simulink model "HLSDem_SetPoint"  (R2016b)
settings: configuration reference "CodeGenConfigSet" (kept outside this file)
values from neighbouring files (symbols this model uses):
  EPM_N_MAX = fi(10000,EngSpeed_rpm)    [init_HLSDem_SetPoint.m]    (also in init_HLSDem_SetPoint_SIL.m)
  HLSDem_dnSetPLoLimHiTrm_C = Calibration.Parameter    [init_HLSDem_SetPoint.m]    (also in init_HLSDem_SetPoint_SIL.m = Simulink.Parameter)
  HLSDem_dnSetPLoLimLoTrm_C = Calibration.Parameter    [init_HLSDem_SetPoint.m]    (also in init_HLSDem_SetPoint_SIL.m = Simulink.Parameter)
  HLSDem_facFdbkCANKick_C = Calibration.Parameter    [init_HLSDem_SetPoint.m]    (also in init_HLSDem_SetPoint_SIL.m = Simulink.Parameter)
  HLSDem_facFdbkDrvKick_C = Calibration.Parameter    [init_HLSDem_SetPoint.m]    (also in init_HLSDem_SetPoint_SIL.m = Simulink.Parameter)
  HLSDem_facFdbkHGG_C = Calibration.Parameter    [init_HLSDem_SetPoint.m]    (also in init_HLSDem_SetPoint_SIL.m = Simulink.Parameter)
  HLSDem_facFdbkLGG_C = Calibration.Parameter    [init_HLSDem_SetPoint.m]    (also in init_HLSDem_SetPoint_SIL.m = Simulink.Parameter)
  HLSDem_facFdbkMaxAcs_C = Calibration.Parameter    [init_HLSDem_SetPoint.m]    (also in init_HLSDem_SetPoint_SIL.m = Simulink.Parameter)
  HLSDem_facFdbkMaxSysErr_C = Calibration.Parameter    [init_HLSDem_SetPoint.m]    (also in init_HLSDem_SetPoint_SIL.m = Simulink.Parameter)
  HLSDem_facFdbkMaxTra_C = Calibration.Parameter    [init_HLSDem_SetPoint.m]    (also in init_HLSDem_SetPoint_SIL.m = Simulink.Parameter)
  HLSDem_facFdbkRed1_C = Calibration.Parameter    [init_HLSDem_SetPoint.m]    (also in init_HLSDem_SetPoint_SIL.m = Simulink.Parameter)
  HLSDem_facFdbkRed2_C = Calibration.Parameter    [init_HLSDem_SetPoint.m]    (also in init_HLSDem_SetPoint_SIL.m = Simulink.Parameter)
  HLSDem_facFdbkRed3_C = Calibration.Parameter    [init_HLSDem_SetPoint.m]    (also in init_HLSDem_SetPoint_SIL.m = Simulink.Parameter)
  HLSDem_facFdbkStrt_C = Calibration.Parameter    [init_HLSDem_SetPoint.m]    (also in init_HLSDem_SetPoint_SIL.m = Simulink.Parameter)
  HLSDem_facFdbkSysDgrt1_C = Calibration.Parameter    [init_HLSDem_SetPoint.m]    (also in init_HLSDem_SetPoint_SIL.m = Simulink.Parameter)
  HLSDem_facFdbkSysDgrt2_C = Calibration.Parameter    [init_HLSDem_SetPoint.m]    (also in init_HLSDem_SetPoint_SIL.m = Simulink.Parameter)
  HLSDem_facFdbkSysDgrt3_C = Calibration.Parameter    [init_HLSDem_SetPoint.m]    (also in init_HLSDem_SetPoint_SIL.m = Simulink.Parameter)
  HLSDem_facSetPLoFlt_C = Calibration.Parameter    [init_HLSDem_SetPoint.m]    (also in init_HLSDem_SetPoint_SIL.m = Simulink.Parameter)
  HLSDem_facTrqHiPT1_C = Calibration.Parameter    [init_HLSDem_SetPoint.m]    (also in init_HLSDem_SetPoint_SIL.m = Simulink.Parameter)
  HLSDem_facTrqLoPT1_C = Calibration.Parameter    [init_HLSDem_SetPoint.m]    (also in init_HLSDem_SetPoint_SIL.m = Simulink.Parameter)
  HLSDem_nHGGSetPHi_C = Calibration.Parameter    [init_HLSDem_SetPoint.m]    (also in init_HLSDem_SetPoint_SIL.m = Simulink.Parameter)
  HLSDem_nKDSetPHi_C = Calibration.Parameter    [init_HLSDem_SetPoint.m]    (also in init_HLSDem_SetPoint_SIL.m = Simulink.Parameter)
  HLSDem_nLGGSetPHi_C = Calibration.Parameter    [init_HLSDem_SetPoint.m]    (also in init_HLSDem_SetPoint_SIL.m = Simulink.Parameter)
  HLSDem_nRed1SetPHi_C = Calibration.Parameter    [init_HLSDem_SetPoint.m]    (also in init_HLSDem_SetPoint_SIL.m = Simulink.Parameter)
  HLSDem_nRed2SetPHi_C = Calibration.Parameter    [init_HLSDem_SetPoint.m]    (also in init_HLSDem_SetPoint_SIL.m = Simulink.Parameter)
  HLSDem_nRed3SetPHi_C = Calibration.Parameter    [init_HLSDem_SetPoint.m]    (also in init_HLSDem_SetPoint_SIL.m = Simulink.Parameter)
  HLSDem_nSel1SetPLo_C = Calibration.Parameter    [init_HLSDem_SetPoint.m]    (also in init_HLSDem_SetPoint_SIL.m = Simulink.Parameter)
  HLSDem_nSel2SetPLo_C = Calibration.Parameter    [init_HLSDem_SetPoint.m]    (also in init_HLSDem_SetPoint_SIL.m = Simulink.Parameter)
  HLSDem_nSel3SetPLo_C = Calibration.Parameter    [init_HLSDem_SetPoint.m]    (also in init_HLSDem_SetPoint_SIL.m = Simulink.Parameter)
  HLSDem_nSetPLoDia_C = Calibration.Parameter    [init_HLSDem_SetPoint.m]    (also in init_HLSDem_SetPoint_SIL.m = Simulink.Parameter)
  HLSDem_nSetPLoDrvAwy_C = Calibration.Parameter    [init_HLSDem_SetPoint.m]    (also in init_HLSDem_SetPoint_SIL.m = Simulink.Parameter)
  HLSDem_nSetPLoIni_CUR = Calibration.Parameter    [init_HLSDem_SetPoint.m]    (also in init_HLSDem_SetPoint_SIL.m = Simulink.Parameter)
  HLSDem_nSetPLoIni_CURX = Calibration.Parameter    [init_HLSDem_SetPoint.m]    (also in init_HLSDem_SetPoint_SIL.m = Simulink.Parameter)
  HLSDem_nSetPLoMax_C = Calibration.Parameter    [init_HLSDem_SetPoint.m]    (also in init_HLSDem_SetPoint_SIL.m = Simulink.Parameter)
  HLSDem_nSetPLoMaxOfs_C = Calibration.Parameter    [init_HLSDem_SetPoint.m]    (also in init_HLSDem_SetPoint_SIL.m = Simulink.Parameter)
  HLSDem_nSetPLoOfsMoF_C = Calibration.Parameter    [init_HLSDem_SetPoint.m]    (also in init_HLSDem_SetPoint_SIL.m = Simulink.Parameter)
  HLSDem_nSetPLoWrm_C = Calibration.Parameter    [init_HLSDem_SetPoint.m]    (also in init_HLSDem_SetPoint_SIL.m = Simulink.Parameter)
  HLSDem_nSpdLowBattUAdd_CUR = Calibration.Parameter    [init_HLSDem_SetPoint.m]    (also in init_HLSDem_SetPoint_SIL.m = Simulink.Parameter)
  HLSDem_nSpdLowBattUAdd_CURX = Calibration.Parameter    [init_HLSDem_SetPoint.m]    (also in init_HLSDem_SetPoint_SIL.m = Simulink.Parameter)
  HLSDem_nSpdLowBattUAddLim_C = Calibration.Parameter    [init_HLSDem_SetPoint.m]    (also in init_HLSDem_SetPoint_SIL.m = Simulink.Parameter)
  HLSDem_nStrtSetPHi_C = Calibration.Parameter    [init_HLSDem_SetPoint.m]    (also in init_HLSDem_SetPoint_SIL.m = Simulink.Parameter)
  HLSDem_nSysDgrtSetPHi_C = Calibration.Parameter    [init_HLSDem_SetPoint.m]    (also in init_HLSDem_SetPoint_SIL.m = Simulink.Parameter)
  HLSDem_rTrqSwt_C = Calibration.Parameter    [init_HLSDem_SetPoint.m]    (also in init_HLSDem_SetPoint_SIL.m = Simulink.Parameter)
  HLSDem_SetPHiRmpSlopeNeg_C = Calibration.Parameter    [init_HLSDem_SetPoint.m]    (also in init_HLSDem_SetPoint_SIL.m = Simulink.Parameter)
  HLSDem_SetPHiRmpSlopePos_C = Calibration.Parameter    [init_HLSDem_SetPoint.m]    (also in init_HLSDem_SetPoint_SIL.m = Simulink.Parameter)
  HLSDem_SetPLoRmpSlopeNeg_C = Calibration.Parameter    [init_HLSDem_SetPoint.m]    (also in init_HLSDem_SetPoint_SIL.m = Simulink.Parameter)
  HLSDem_SetPLoRmpSlopePos_C = Calibration.Parameter    [init_HLSDem_SetPoint.m]    (also in init_HLSDem_SetPoint_SIL.m = Simulink.Parameter)
  HLSDem_SetPLoTipInRmpSlopeNeg_C = Calibration.Parameter    [init_HLSDem_SetPoint.m]    (also in init_HLSDem_SetPoint_SIL.m = Simulink.Parameter)
  HLSDem_SetPLoTipInRmpSlopePos_C = Calibration.Parameter    [init_HLSDem_SetPoint.m]    (also in init_HLSDem_SetPoint_SIL.m = Simulink.Parameter)
  HLSDem_stSetPLoFlt_C = Calibration.Parameter    [init_HLSDem_SetPoint.m]    (also in init_HLSDem_SetPoint_SIL.m = Simulink.Parameter)
  HLSDem_stSpdSel_C = Calibration.Parameter    [init_HLSDem_SetPoint.m]    (also in init_HLSDem_SetPoint_SIL.m = Simulink.Parameter)
  HLSDem_stSysDgrtSetPHi_C = Calibration.Parameter    [init_HLSDem_SetPoint.m]    (also in init_HLSDem_SetPoint_SIL.m = Simulink.Parameter)
  HLSDem_swtDisblVehIfcSetPHi_C = Calibration.Parameter    [init_HLSDem_SetPoint.m]    (also in init_HLSDem_SetPoint_SIL.m = Simulink.Parameter)
  HLSDem_swtEnaPTO_C = Calibration.Parameter    [init_HLSDem_SetPoint.m]    (also in init_HLSDem_SetPoint_SIL.m = Simulink.Parameter)
  HLSDem_swtMode_C = Calibration.Parameter    [init_HLSDem_SetPoint.m]    (also in init_HLSDem_SetPoint_SIL.m = Simulink.Parameter)
  HLSDem_swtTempSel_C = Calibration.Parameter    [init_HLSDem_SetPoint.m]    (also in init_HLSDem_SetPoint_SIL.m = Simulink.Parameter)
  HLSDem_swtTrqHiSel_C = Calibration.Parameter    [init_HLSDem_SetPoint.m]    (also in init_HLSDem_SetPoint_SIL.m = Simulink.Parameter)
  HLSDem_swtTrqLoSel_C = Calibration.Parameter    [init_HLSDem_SetPoint.m]    (also in init_HLSDem_SetPoint_SIL.m = Simulink.Parameter)
  HLSDem_tDflSetPLo_C = Calibration.Parameter    [init_HLSDem_SetPoint.m]    (also in init_HLSDem_SetPoint_SIL.m = Simulink.Parameter)
  HLSDem_tiMaxIncrSetPLo_C = Calibration.Parameter    [init_HLSDem_SetPoint.m]    (also in init_HLSDem_SetPoint_SIL.m = Simulink.Parameter)
  HLSDem_tiSpdLowBattUAdd_C = Calibration.Parameter    [init_HLSDem_SetPoint.m]    (also in init_HLSDem_SetPoint_SIL.m = Simulink.Parameter)
  HLSDem_tiStrtCEngDsT_CUR = Calibration.Parameter    [init_HLSDem_SetPoint.m]    (also in init_HLSDem_SetPoint_SIL.m = Simulink.Parameter)
  HLSDem_tiStrtCEngDsT_CURX = Calibration.Parameter    [init_HLSDem_SetPoint.m]    (also in init_HLSDem_SetPoint_SIL.m = Simulink.Parameter)
  HLSDem_tiStrtEngOil_CUR = Calibration.Parameter    [init_HLSDem_SetPoint.m]    (also in init_HLSDem_SetPoint_SIL.m = Simulink.Parameter)
  HLSDem_tiStrtEngOil_CURX = Calibration.Parameter    [init_HLSDem_SetPoint.m]    (also in init_HLSDem_SetPoint_SIL.m = Simulink.Parameter)
  HLSDem_tThresDisbl_C = Calibration.Parameter    [init_HLSDem_SetPoint.m]    (also in init_HLSDem_SetPoint_SIL.m = Simulink.Parameter)
  HLSDem_tThresEna_C = Calibration.Parameter    [init_HLSDem_SetPoint.m]    (also in init_HLSDem_SetPoint_SIL.m = Simulink.Parameter)
  HLSDem_volSpdAddHi_C = Calibration.Parameter    [init_HLSDem_SetPoint.m]    (also in init_HLSDem_SetPoint_SIL.m = Simulink.Parameter)
  HLSDem_volSpdAddLo_C = Calibration.Parameter    [init_HLSDem_SetPoint.m]    (also in init_HLSDem_SetPoint_SIL.m = Simulink.Parameter)
  HndBrk_stDebVal_C = Calibration.Parameter    [init_HLSDem_SetPoint.m]    (also in init_HLSDem_SetPoint_SIL.m = Simulink.Parameter)
  SigTst_nSetPHi_C = Calibration.Parameter    [init_HLSDem_SetPoint.m]    (also in init_HLSDem_SetPoint_SIL.m = Simulink.Parameter)
  SigTst_nSetPLo_C = Calibration.Parameter    [init_HLSDem_SetPoint.m]    (also in init_HLSDem_SetPoint_SIL.m = Simulink.Parameter)
  SigTst_swtSetPHi_C = Calibration.Parameter    [init_HLSDem_SetPoint.m]    (also in init_HLSDem_SetPoint_SIL.m = Simulink.Parameter)
  SigTst_swtSetPLo_C = Calibration.Parameter    [init_HLSDem_SetPoint.m]    (also in init_HLSDem_SetPoint_SIL.m = Simulink.Parameter)
undefined symbols (not defined in the file or in its folder): CEngDst_switch_conv, CEngDsT_tTransf_CURX, EngState_conv, HLSDem_SetPoint_DT, StSys_StrtState_conv, Switch_conv
libraries: CXLib x13, simulink x3
(part 2 of 2)

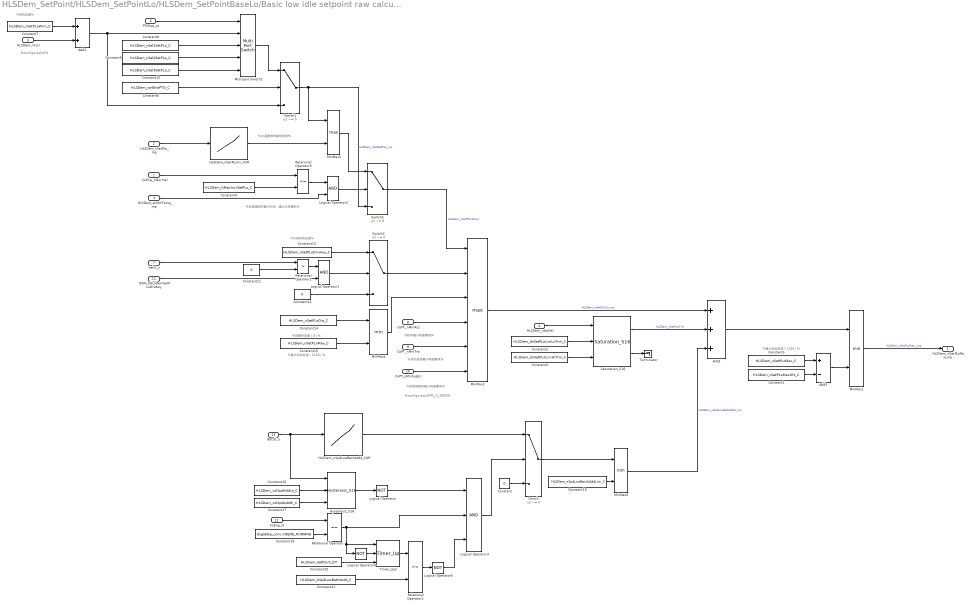
== system HLSDem_SetPoint/HLSDem_SetPointLo/HLSDem_SetPointBaseLo/Basic low idle setpoint raw calculation ==
  note: %最大目标怠速（1100）%
  note: %故障时怠速（0）%
  note: %configured=EPM_N_ZERO%
  note: %怠速增加的最大时间，确认已经暖机%
  note: %热机怠速%
  note: %最大目标怠速（1100）%
  note: %行驶时的怠速%
  note: %附件最小转速需求%
  note: %系统错误时最小转速需求%
  note: %传动系统最小转速需求%
  note: %configured=0%
  note: %水温要求的最低转速%
  CoEng_tiNormal : Inport
  HLSDem_tSetPLo_mp : Inport  Port=2
  HLSDem_stStrtTemp_mp : Inport  Port=3
  HLSDem_nAdjVal : Inport  Port=4
  HLSDem_nIncr : Inport  Port=5
  PTOSwt_st : Inport  Port=6
  VehV_v : Inport  Port=7
  CoPT_nMinAcs : Inport  Port=8
  CoPT_nMinTra : Inport  Port=9
  CoPT_nMinSysErr : Inport  Port=10
  DSM_bHLSDemSetPLoDrvAwy : Inport  Port=11
  CoEng_st : Inport  Port=12
  BattU_u : Inport  Tag=mv  Description=Battery voltage  Port=13  OutMin=0  OutMax=50000  OutDataTypeStr=Battery_mv
  Add1 : Sum  Inputs=+++  SaturateOnIntegerOverflow=on  InputSameDT=on
  Add2 : Sum  SaturateOnIntegerOverflow=on  InputSameDT=on
  Add3 : Sum  Inputs=+-  SaturateOnIntegerOverflow=on  InputSameDT=on
  Constant : Constant  Value=0  OutDataTypeStr=Inherit: Inherit via back propagation
  Constant1 : Constant  Value=HLSDem_nSetPLoMaxOfs_C
  Constant10 : Constant  Value=HLSDem_nSel3SetPLo_C
  Constant11 : Constant  Value=0  OutDataTypeStr=Inherit: Inherit via back propagation
  Constant12 : Constant  Value=0  OutDataTypeStr=Inherit: Inherit via back propagation
  Constant13 : Constant  Value=HLSDem_nSetPLoDrvAwy_C
  Constant14 : Constant  Value=HLSDem_nSetPLoDia_C
  Constant15 : Constant  Value=HLSDem_nSetPLoMax_C
  Constant16 : Constant  Value=HLSDem_volSpdAddLo_C
  Constant17 : Constant  Value=HLSDem_volSpdAddHi_C
  Constant18 : Constant  Value=EngState_conv.COENG_RUNNING
  Constant19 : Constant  Value=HLSDem_nSpdLowBattUAddLim_C
  Constant2 : Constant  Value=HLSDem_dnSetPLoLimLoTrm_C  SampleTime=-1
  Constant20 : Constant  Value=HLSDem_SetPoint_DT  OutDataTypeStr=Inherit: Inherit via back propagation
  Constant21 : Constant  Value=HLSDem_tiSpdLowBattUAdd_C
  Constant3 : Constant  Value=HLSDem_dnSetPLoLimHiTrm_C  SampleTime=-1
  Constant4 : Constant  Value=HLSDem_tiMaxIncrSetPLo_C
  Constant5 : Constant  Value=HLSDem_nSetPLoMax_C
  Constant6 : Constant  Value=HLSDem_swtEnaPTO_C
  Constant7 : Constant  Value=HLSDem_nSetPLoWrm_C
  Constant8 : Constant  Value=HLSDem_nSel1SetPLo_C
  Constant9 : Constant  Value=HLSDem_nSel2SetPLo_C
  HLSDem_nSetPLoIni_CUR : Lookup_n-D  DialogController=Simulink.DDGSource  NumberOfTableDimensions=1  BreakpointsForDimension1=HLSDem_nSetPLoIni_CURX  BreakpointsForDimension2=CEngDsT_tTransf_CURX  IndexSearchMethod=Linear search  BeginIndexSearchUsingPreviousIndexResult=on  Table=HLSDem_nSetPLoIni_CUR  ExtrapMethod=Clip  UseLastTableValue=on  InternalRulePriority=Speed  OutDataTypeStr=Inherit: Inherit via back propagation  SaturateOnIntegerOverflow=on
  HLSDem_nSpdLowBattUAdd_CUR : Lookup_n-D  NumberOfTableDimensions=1  BreakpointsForDimension1=HLSDem_nSpdLowBattUAdd_CURX  IndexSearchMethod=Linear search  BeginIndexSearchUsingPreviousIndexResult=on  Table=HLSDem_nSpdLowBattUAdd_CUR  ExtrapMethod=Clip  UseLastTableValue=on  InternalRulePriority=Speed  OutDataTypeStr=Inherit: Inherit from 'Table data'  RndMeth=Simplest  SaturateOnIntegerOverflow=on
  Hysteresis_S16 : CXLib/Hysteresis_S16
  Logical Operator : Logic  Operator=NOT  AllPortsSameDT=off  OutDataTypeStr=boolean
  Logical Operator1 : Logic  OutDataTypeStr=boolean
  Logical Operator2 : Logic  OutDataTypeStr=boolean
  Logical Operator3 : Logic  Inputs=3  AllPortsSameDT=off  OutDataTypeStr=boolean
  Logical Operator4 : Logic  Operator=NOT  AllPortsSameDT=off  OutDataTypeStr=boolean
  Logical Operator5 : Logic  Operator=NOT  AllPortsSameDT=off  OutDataTypeStr=boolean
  MinMax1 : MinMax  Inputs=2  SaturateOnIntegerOverflow=on  InputSameDT=on
  MinMax2 : MinMax  RequirementInfo={'other' 'HLSDem_SetPointLo_requirements.docx' '@Simulink_requirement_item_20' 'true' '选择目标怠速' '' } %GIDa_1dec2fce_e581_44b4_8998_b8679ade50a4  Function=max  Inputs=6  SaturateOnIntegerOverflow=on  InputSameDT=on
  MinMax3 : MinMax  Function=max  Inputs=2  SaturateOnIntegerOverflow=on  InputSameDT=on
  MinMax4 : MinMax  Inputs=2  SaturateOnIntegerOverflow=on  InputSameDT=on
  MinMax5 : MinMax  Inputs=2  SaturateOnIntegerOverflow=on
  Multiport Switch2 : MultiPortSwitch  DataPortOrder=Zero-based contiguous  Inputs=4  DiagnosticForDefault=Warning  SaturateOnIntegerOverflow=on  InputSameDT=on
  Relational Operator : RelationalOperator  Operator===  OutDataTypeStr=boolean  RndMeth=Simplest
  Relational Operator1 : RelationalOperator  Operator=>  OutDataTypeStr=boolean  RndMeth=Nearest  InputSameDT=on
  Relational Operator2 : RelationalOperator  OutDataTypeStr=boolean  RndMeth=Simplest  InputSameDT=on
  Relational Operator9 : RelationalOperator  Operator=<=  OutDataTypeStr=boolean  RndMeth=Nearest  InputSameDT=on
  Saturation_S16 : CXLib/Saturation_S16  RequirementInfo={'other' 'HLSDem_SetPointLo_requirements.docx' '@Simulink_requirement_item_21' 'true' '目标怠速调整及限制' '' } %GIDa_15563632_a417_4a1b_8a84_0934a39ef2cd
  Switch : Switch  Criteria=u2 ~= 0  InputSameDT=on
  Switch1 : Switch  Criteria=u2 ~= 0  SaturateOnIntegerOverflow=on  InputSameDT=on
  Switch2 : Switch  Criteria=u2 ~= 0  SaturateOnIntegerOverflow=on  InputSameDT=on
  Switch5 : Switch  RequirementInfo={'other' 'HLSDem_SetPointLo_requirements.docx' '@Simulink_requirement_item_19' 'true' '目标怠速自动增加功能' '' } %GIDa_4e10bb43_f23f_486a_82bf_1b96970b13ef  Criteria=u2 ~= 0  SaturateOnIntegerOverflow=on  InputSameDT=on
  Terminator : Terminator
  Timer_Up2 : CXLib/Timer_Up
  HLSDem_nSetPLoRaw_mp : Outport
  wires:
  Constant11/1 -> Relational Operator1/2
  CoPT_nMinSysErr/1 -> MinMax2/6
  CoPT_nMinTra/1 -> MinMax2/5
  CoPT_nMinAcs/1 -> MinMax2/4
  MinMax4/1 -> MinMax2/3
  Constant15/1 -> MinMax4/2
  Constant14/1 -> MinMax4/1
  Switch2/1 -> MinMax2/2
  Constant13/1 -> Switch2/1
  Constant12/1 -> Switch2/3
  DSM_bHLSDemSetPLoDrvAwy/1 -> Logical Operator1/2
  Relational Operator1/1 -> Logical Operator1/1
  VehV_v/1 -> Relational Operator1/1
  Logical Operator1/1 -> Switch2/2
  Switch5/1 -> MinMax2/1  "HLSDem_nSetPLoTemp"
  MinMax3/1 -> Switch5/1
  Constant10/1 -> Multiport Switch2/5
  Constant9/1 -> Multiport Switch2/4
  Constant8/1 -> Multiport Switch2/3
  PTOSwt_st/1 -> Multiport Switch2/1
  Multiport Switch2/1 -> Switch1/1
  HLSDem_nIncr/1 -> Add2/2
  Constant7/1 -> Add2/1
  Add2/1 -> Multiport Switch2/2, Switch1/3
  Constant6/1 -> Switch1/2
  Switch1/1 -> MinMax3/1, Switch5/3  "HLSDem_nSelSetPLo_mp"
  HLSDem_tSetPLo_mp/1 -> HLSDem_nSetPLoIni_CUR/1
  HLSDem_nSetPLoIni_CUR/1 -> MinMax3/2
  HLSDem_stStrtTemp_mp/1 -> Logical Operator2/2
  CoEng_tiNormal/1 -> Relational Operator9/1
  Constant4/1 -> Relational Operator9/2
  Relational Operator9/1 -> Logical Operator2/1
  Logical Operator2/1 -> Switch5/2
  MinMax2/1 -> Add1/1  "HLSDem_nSetPLoCo_mp"
  HLSDem_nAdjVal/1 -> Saturation_S16/1
  Constant3/1 -> Saturation_S16/3
  Constant2/1 -> Saturation_S16/2
  Saturation_S16/2 -> Terminator/1
  Saturation_S16/1 -> Add1/2  "HLSDem_nSetPLoTrm"
  Add1/1 -> MinMax1/1
  MinMax1/1 -> HLSDem_nSetPLoRaw_mp/1  "HLSDem_nSetPLoRaw_mp"
  Constant1/1 -> Add3/2
  Constant5/1 -> Add3/1
  Add3/1 -> MinMax1/2
  BattU_u/1 -> Hysteresis_S16/1, HLSDem_nSpdLowBattUAdd_CUR/1
  HLSDem_nSpdLowBattUAdd_CUR/1 -> Switch/1
  Hysteresis_S16/1 -> Logical Operator/1
  Constant/1 -> Switch/3
  Constant16/1 -> Hysteresis_S16/2
  Constant17/1 -> Hysteresis_S16/3
  CoEng_st/1 -> Relational Operator/1
  Constant18/1 -> Relational Operator/2
  Logical Operator/1 -> Logical Operator3/1
  Relational Operator/1 -> Logical Operator3/2, Timer_Up2/1, Logical Operator4/1
  Logical Operator3/1 -> Switch/2
  Switch/1 -> MinMax5/1
  MinMax5/1 -> Add1/3  "HLSDem_nSpdLowBattUAdd_mp"
  Constant19/1 -> MinMax5/2
  Logical Operator4/1 -> Timer_Up2/2
  Constant20/1 -> Timer_Up2/3
  Timer_Up2/1 -> Relational Operator2/1
  Constant21/1 -> Relational Operator2/2
  Relational Operator2/1 -> Logical Operator5/1
  Logical Operator5/1 -> Logical Operator3/3

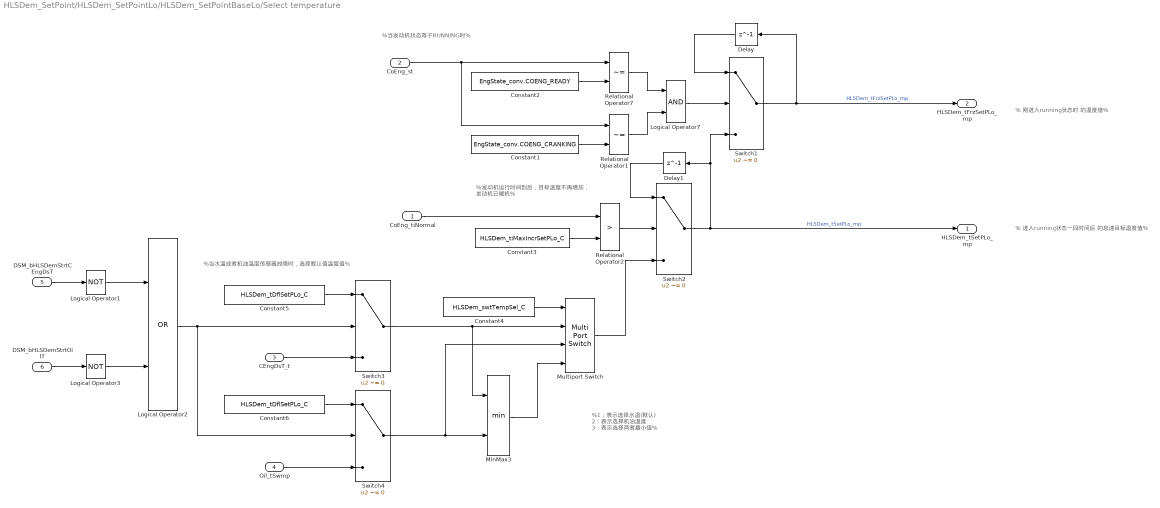
== system HLSDem_SetPoint/HLSDem_SetPointLo/HLSDem_SetPointBaseLo/Select temperature ==
  note: %当水温或者机油温度传感器故障时，选择默认值温度值%
  note: %当发动机状态等于RUNNING时%
  note: % 刚进入running状态时 的温度值%
  note: % 进入running状态一段时间后 的怠速目标温度值%
  note: %1：表示选择水温(默认)
      | 2：表示选择机油温度
      | 3：表示选择两者最小值%
  note: %发动机运行时间到后，目标温度不再增加，
      | 发动机已暖机%
  CoEng_tiNormal : Inport
  CoEng_st : Inport  Port=2
  CEngDsT_t : Inport  Port=3
  Oil_tSwmp : Inport  Port=4
  DSM_bHLSDemStrtCEngDsT : Inport  Port=5
  DSM_bHLSDemStrtOilT : Inport  Port=6
  Constant1 : Constant  Value=EngState_conv.COENG_CRANKING
  Constant2 : Constant  Value=EngState_conv.COENG_READY
  Constant3 : Constant  Value=HLSDem_tiMaxIncrSetPLo_C
  Constant4 : Constant  Value=HLSDem_swtTempSel_C
  Constant5 : Constant  Value=HLSDem_tDflSetPLo_C
  Constant6 : Constant  Value=HLSDem_tDflSetPLo_C
  Delay : Delay  DelayLength=1  InitialCondition=0
  Delay1 : Delay  DelayLength=1  InitialCondition=0
  Logical Operator1 : Logic  Operator=NOT  AllPortsSameDT=off  OutDataTypeStr=boolean
  Logical Operator2 : Logic  Operator=OR  OutDataTypeStr=boolean
  Logical Operator3 : Logic  Operator=NOT  AllPortsSameDT=off  OutDataTypeStr=boolean
  Logical Operator7 : Logic  OutDataTypeStr=boolean
  MinMax3 : MinMax  Inputs=2  SaturateOnIntegerOverflow=on  InputSameDT=on
  Multiport Switch : MultiPortSwitch  DiagnosticForDefault=Warning  SaturateOnIntegerOverflow=on  InputSameDT=on
  Relational Operator1 : RelationalOperator  Operator=~=  OutDataTypeStr=boolean  RndMeth=Nearest  InputSameDT=on
  Relational Operator2 : RelationalOperator  Operator=>  OutDataTypeStr=boolean  RndMeth=Nearest  InputSameDT=on
  Relational Operator7 : RelationalOperator  Operator=~=  OutDataTypeStr=boolean  RndMeth=Nearest  InputSameDT=on
  Switch{1..4} (4 alike) : Switch  Criteria=u2 ~= 0  SaturateOnIntegerOverflow=on  InputSameDT=on
  HLSDem_tSetPLo_mp : Outport
  HLSDem_tFrzSetPLo_mp : Outport  Port=2
  wires:
  Logical Operator7/1 -> Switch1/2
  MinMax3/1 -> Multiport Switch/4
  Switch4/1 -> MinMax3/2, Multiport Switch/3
  Oil_tSwmp/1 -> Switch4/3
  Constant6/1 -> Switch4/1
  Switch3/1 -> Multiport Switch/2, MinMax3/1
  CEngDsT_t/1 -> Switch3/3
  Constant5/1 -> Switch3/1
  Logical Operator3/1 -> Logical Operator2/2
  DSM_bHLSDemStrtCEngDsT/1 -> Logical Operator1/1
  Logical Operator2/1 -> Switch3/2, Switch4/2
  Logical Operator1/1 -> Logical Operator2/1
  Constant4/1 -> Multiport Switch/1
  Multiport Switch/1 -> Switch2/3
  Delay1/1 -> Switch2/1
  Constant3/1 -> Relational Operator2/2
  Relational Operator2/1 -> Switch2/2
  CoEng_tiNormal/1 -> Relational Operator2/1
  Switch2/1 -> Delay1/1, Switch1/3, HLSDem_tSetPLo_mp/1  "HLSDem_tSetPLo_mp"
  Delay/1 -> Switch1/1
  Relational Operator1/1 -> Logical Operator7/2
  Relational Operator7/1 -> Logical Operator7/1
  Constant1/1 -> Relational Operator1/2
  Constant2/1 -> Relational Operator7/2
  CoEng_st/1 -> Relational Operator7/1, Relational Operator1/1
  Switch1/1 -> Delay/1, HLSDem_tFrzSetPLo_mp/1  "HLSDem_tFrzSetPLo_mp"
  DSM_bHLSDemStrtOilT/1 -> Logical Operator3/1

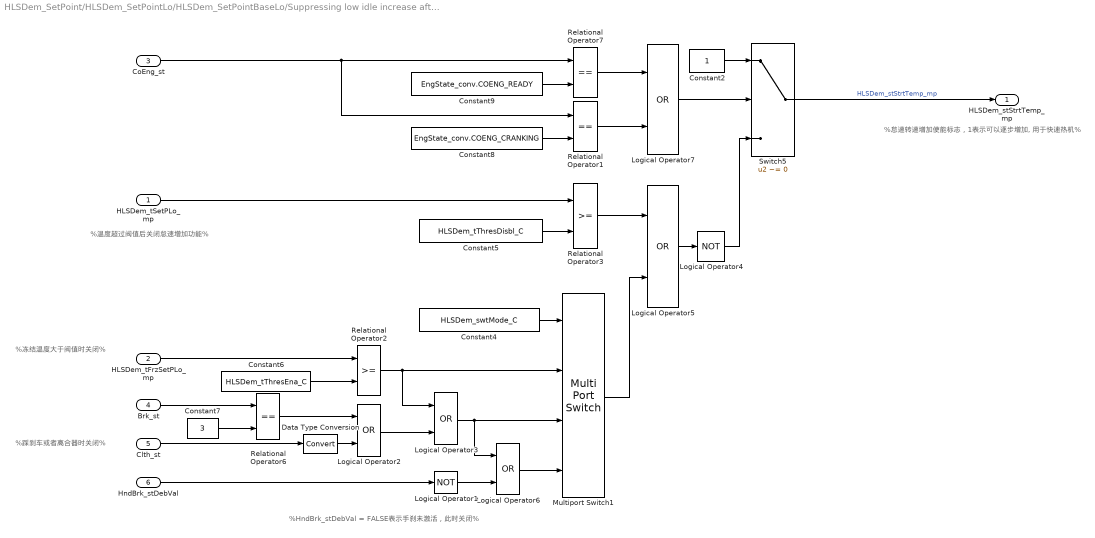
== system HLSDem_SetPoint/HLSDem_SetPointLo/HLSDem_SetPointBaseLo/Suppressing low idle increase after start ==
  note: %HndBrk_stDebVal = FALSE表示手刹未激活，此时关闭%
  note: %怠速转速增加使能标志，1表示可以逐步增加,
      | 用于快速热机%
  note: %温度超过阀值后关闭怠速增加功能%
  note: %冻结温度大于阀值时关闭%
  note: %踩刹车或者离合器时关闭%
  HLSDem_tSetPLo_mp : Inport
  HLSDem_tFrzSetPLo_mp : Inport  Port=2
  CoEng_st : Inport  Port=3
  Brk_st : Inport  Port=4
  Clth_st : Inport  Port=5
  HndBrk_stDebVal : Inport  Port=6
  Constant2 : Constant  OutDataTypeStr=Inherit: Inherit via back propagation
  Constant4 : Constant  Value=HLSDem_swtMode_C
  Constant5 : Constant  Value=HLSDem_tThresDisbl_C
  Constant6 : Constant  Value=HLSDem_tThresEna_C
  Constant7 : Constant  Value=3  OutDataTypeStr=Inherit: Inherit via back propagation
  Constant8 : Constant  Value=EngState_conv.COENG_CRANKING
  Constant9 : Constant  Value=EngState_conv.COENG_READY
  Data Type Conversion : DataTypeConversion
  Logical Operator1 : Logic  Operator=NOT  AllPortsSameDT=off  OutDataTypeStr=boolean
  Logical Operator{2..3,5..7} (5 alike) : Logic  Operator=OR  OutDataTypeStr=boolean
  Logical Operator4 : Logic  Operator=NOT  AllPortsSameDT=off  OutDataTypeStr=boolean
  Multiport Switch1 : MultiPortSwitch  DiagnosticForDefault=Warning  SaturateOnIntegerOverflow=on  InputSameDT=on
  Relational Operator1 : RelationalOperator  Operator===  OutDataTypeStr=boolean  RndMeth=Nearest  InputSameDT=on
  Relational Operator2 : RelationalOperator  OutDataTypeStr=boolean  RndMeth=Nearest  InputSameDT=on
  Relational Operator3 : RelationalOperator  OutDataTypeStr=boolean  RndMeth=Nearest  InputSameDT=on
  Relational Operator6 : RelationalOperator  Operator===  OutDataTypeStr=boolean  RndMeth=Nearest  InputSameDT=on
  Relational Operator7 : RelationalOperator  Operator===  OutDataTypeStr=boolean  RndMeth=Nearest  InputSameDT=on
  Switch5 : Switch  Criteria=u2 ~= 0  SaturateOnIntegerOverflow=on  InputSameDT=on
  HLSDem_stStrtTemp_mp : Outport
  wires:
  Data Type Conversion/1 -> Logical Operator2/2
  CoEng_st/1 -> Relational Operator7/1, Relational Operator1/1
  Switch5/1 -> HLSDem_stStrtTemp_mp/1  "HLSDem_stStrtTemp_mp"
  Relational Operator6/1 -> Logical Operator2/1
  HndBrk_stDebVal/1 -> Logical Operator1/1
  Logical Operator1/1 -> Logical Operator6/2
  Logical Operator6/1 -> Multiport Switch1/4
  Clth_st/1 -> Data Type Conversion/1
  Brk_st/1 -> Relational Operator6/1
  Constant7/1 -> Relational Operator6/2
  Logical Operator2/1 -> Logical Operator3/2
  Logical Operator3/1 -> Multiport Switch1/3, Logical Operator6/1
  Constant6/1 -> Relational Operator2/2
  HLSDem_tFrzSetPLo_mp/1 -> Relational Operator2/1
  Relational Operator2/1 -> Multiport Switch1/2, Logical Operator3/1
  Constant4/1 -> Multiport Switch1/1
  Multiport Switch1/1 -> Logical Operator5/2
  Relational Operator3/1 -> Logical Operator5/1
  Constant5/1 -> Relational Operator3/2
  HLSDem_tSetPLo_mp/1 -> Relational Operator3/1
  Logical Operator5/1 -> Logical Operator4/1
  Logical Operator4/1 -> Switch5/3
  Constant8/1 -> Relational Operator1/2
  Logical Operator7/1 -> Switch5/2
  Relational Operator1/1 -> Logical Operator7/2
  Relational Operator7/1 -> Logical Operator7/1
  Constant9/1 -> Relational Operator7/2
  Constant2/1 -> Switch5/1

== system HLSDem_SetPoint/HLSDem_SetPointLo/HLSDem_SetPointBaseLo/Basic low idle setpoint calculation/Fiter state determination ==
  note: %3:Step
      | 2：经过PT1滤波
      | 1：经过斜坡(Tipin)
      | 0：经过斜坡功能%
  Constant11 : Constant  Value=HLSDem_stSetPLoFlt_C  SampleTime=-1
  HLSDem_stSetPLoFlt_mp : Outport
  wires:
  Constant11/1 -> HLSDem_stSetPLoFlt_mp/1

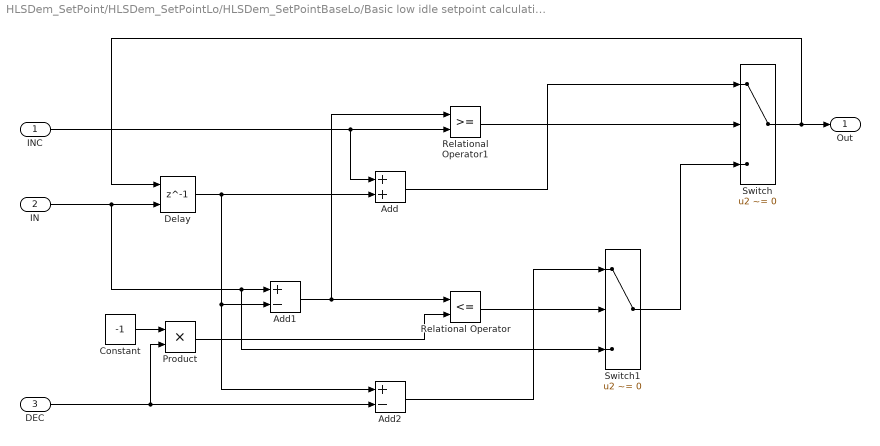
== system HLSDem_SetPoint/HLSDem_SetPointLo/HLSDem_SetPointBaseLo/Basic low idle setpoint calculation/RAMP1 ==
  INC : Inport
  IN : Inport  Port=2
  DEC : Inport  Port=3
  Add : Sum  InputSameDT=on
  Add1 : Sum  Inputs=+-  InputSameDT=on
  Add2 : Sum  Inputs=+-  InputSameDT=on
  Constant : Constant  Value=-1  OutDataTypeStr=Inherit: Inherit via back propagation
  Delay : Delay  DelayLength=1  InitialConditionSource=Input port
      settings: InputPortMap=u0,p4
  Product : Product  OutDataTypeStr=Inherit: Inherit via back propagation  InputSameDT=on
  Relational Operator : RelationalOperator  Operator=<=  OutDataTypeStr=boolean  RndMeth=Simplest  InputSameDT=on
  Relational Operator1 : RelationalOperator  OutDataTypeStr=boolean  RndMeth=Simplest
  Switch : Switch  Criteria=u2 ~= 0
  Switch1 : Switch  Criteria=u2 ~= 0
  Out : Outport
  wires:
  IN/1 -> Switch1/3, Add1/1, Delay/2
  Delay/1 -> Add2/1, Add1/2, Add/2
  Add1/1 -> Relational Operator1/1, Relational Operator/1
  INC/1 -> Add/1, Relational Operator1/2
  Relational Operator1/1 -> Switch/2
  Add/1 -> Switch/1
  Switch/1 -> Delay/1, Out/1
  Relational Operator/1 -> Switch1/2
  Switch1/1 -> Switch/3
  Constant/1 -> Product/1
  DEC/1 -> Product/2, Add2/2
  Product/1 -> Relational Operator/2
  Add2/1 -> Switch1/1

== system HLSDem_SetPoint/HLSDem_SetPointLo/HLSDem_SetPointBaseLo/Basic low idle setpoint calculation/RAMP2 ==
  INC : Inport
  IN : Inport  Port=2
  DEC : Inport  Port=3
  Add : Sum  InputSameDT=on
  Add1 : Sum  Inputs=+-
  Add2 : Sum  Inputs=+-  InputSameDT=on
  Constant : Constant  Value=-1  OutDataTypeStr=Inherit: Inherit via back propagation
  Delay : Delay  DelayLength=1  InitialConditionSource=Input port
      settings: InputPortMap=u0,p4
  Product : Product  OutDataTypeStr=Inherit: Inherit via back propagation
  Relational Operator : RelationalOperator  Operator=<=  OutDataTypeStr=boolean  RndMeth=Simplest  InputSameDT=on
  Relational Operator1 : RelationalOperator  OutDataTypeStr=boolean  RndMeth=Simplest  InputSameDT=on
  Switch : Switch  Criteria=u2 ~= 0
  Switch1 : Switch  Criteria=u2 ~= 0
  Out : Outport
  wires:
  IN/1 -> Switch1/3, Add1/1, Delay/2
  Delay/1 -> Add2/1, Add1/2, Add/2
  Add1/1 -> Relational Operator1/1, Relational Operator/1
  INC/1 -> Add/1, Relational Operator1/2
  Relational Operator1/1 -> Switch/2
  Add/1 -> Switch/1
  Switch/1 -> Delay/1, Out/1
  Relational Operator/1 -> Switch1/2
  Switch1/1 -> Switch/3
  Constant/1 -> Product/1
  DEC/1 -> Product/2, Add2/2
  Product/1 -> Relational Operator/2
  Add2/1 -> Switch1/1
